simulink model "ExempleSimulink_7"  (R2019b)
settings: Solver=VariableStepAuto  StartTime=0.0  StopTime=10  MaxStep=1/2000  RelTol=1e-3
settings Model: Creator=eric  LastModifiedBy=maxim
settings DataIOCC: ReturnWorkspaceOutputs=off
settings DebuggingCC: ArithmeticOperatorsInVariantConditions=warning
settings SFSimCC: SimUseLocalCustomCode=off  CustomCodeUndefinedFunction=UseInterfaceOnly
settings RTWCC: RTWUseLocalCustomCode=off

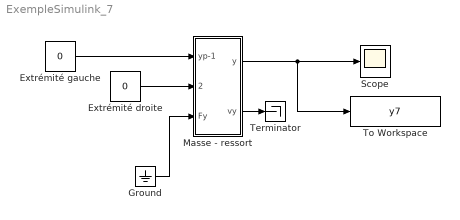
== system ExempleSimulink_7 ==
  Extrémité droite : Constant  Value=0
  Extrémité gauche : Constant  Value=0
  Ground : Ground
  Masse - ressort : Subsystem  mask{m=0.00325, k=155.23, b=0.001, pos_ini=0.01, v_ini=0}
      mask prompts: m "Masse"; k "Force rappel d'un ressort"; b "Frottement"; pos_ini "Position initiale"; v_ini "Vitesse initiale"
  Scope : Scope
  Terminator : Terminator
  To Workspace : ToWorkspace  VariableName=y7  SaveFormat=Timeseries  SampleTime=-1
  wires:
  Masse - ressort/2(vy) -> Terminator/1
  Ground/1 -> Masse - ressort/3(Fy)
  Extrémité droite/1 -> Masse - ressort/2(yp+1)
  Masse - ressort/1(y) -> To Workspace/1, Scope/1
  Extrémité gauche/1 -> Masse - ressort/1(yp-1)

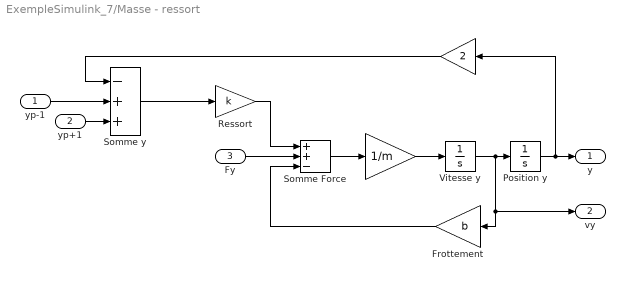
== system ExempleSimulink_7/Masse - ressort ==
  yp-1 : Inport
  yp+1 : Inport  Port=2
  Fy : Inport  Port=3
  " " : Gain  Gain=2  SaturateOnIntegerOverflow=on  OutDataTypeStr=Inherit: Same as input  ParamDataTypeStr=Inherit: Same as input
  "  " : Gain  Gain=1/m  SaturateOnIntegerOverflow=on  OutDataTypeStr=Inherit: Same as input  ParamDataTypeStr=Inherit: Same as input
  Frottement : Gain  Gain=b  SaturateOnIntegerOverflow=on  OutDataTypeStr=Inherit: Same as input  ParamDataTypeStr=Inherit: Same as input
  Position y : Integrator  InitialCondition=pos_ini
  Ressort : Gain  Gain=k  SaturateOnIntegerOverflow=on  OutDataTypeStr=Inherit: Same as input  ParamDataTypeStr=Inherit: Same as input
  Somme Force : Sum  Inputs=++-  SaturateOnIntegerOverflow=on  InputSameDT=on  OutDataTypeStr=Inherit: Same as first input
  Somme y : Sum  Inputs=-++  SaturateOnIntegerOverflow=on  InputSameDT=on  OutDataTypeStr=Inherit: Same as first input
  Vitesse y : Integrator  InitialCondition=v_ini
  y : Outport  VectorParamsAs1DForOutWhenUnconnected=off
  vy : Outport  Port=2  VectorParamsAs1DForOutWhenUnconnected=off
  wires:
  Position y/1 -> " "/1, y/1
  Vitesse y/1 -> Position y/1, Frottement/1, vy/1
  "  "/1 -> Vitesse y/1
  Somme Force/1 -> "  "/1
  Ressort/1 -> Somme Force/1
  Somme y/1 -> Ressort/1
  Frottement/1 -> Somme Force/3
  Fy/1 -> Somme Force/2
  yp+1/1 -> Somme y/3
  yp-1/1 -> Somme y/2
  " "/1 -> Somme y/1
